simulink model "equ_diff"  (R2014a)
settings: Solver=ode45  StartTime=0.0  StopTime=10  RelTol=1e-3
values from neighbouring files (symbols this model uses):
  g = 9.81    [boucle_ferme.m]    (also in commande.m; var.m = 9.8)
  lp = 0.3    [boucle_ferme.m]    (also in commande.m; var.m = 0.2)
  mc = 0.5    [boucle_ferme.m]    (also in commande.m; var.m = 0.1)
  mp = 0.2    [boucle_ferme.m]    (also in commande.m; var.m)
settings Model: Creator=yassin  LastModifiedBy=yassin
settings DebuggingCC: UnderspecifiedInitializationDetection=Classic  StateNameClashWarn=warning

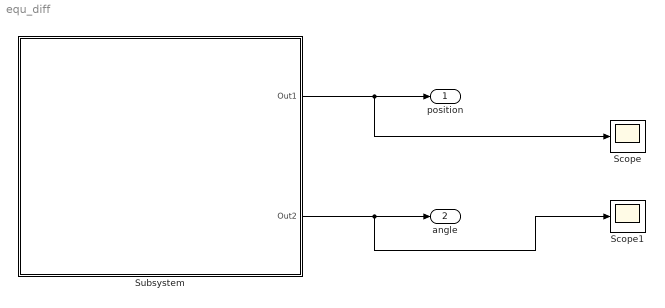
== system equ_diff ==
  Scope : Scope
  Scope1 : Scope
  Subsystem : Subsystem
  position : Outport
  angle : Outport  Port=2
  wires:
  Subsystem/1(Out1) -> Scope/1, position/1
  Subsystem/2(Out2) -> Scope1/1, angle/1

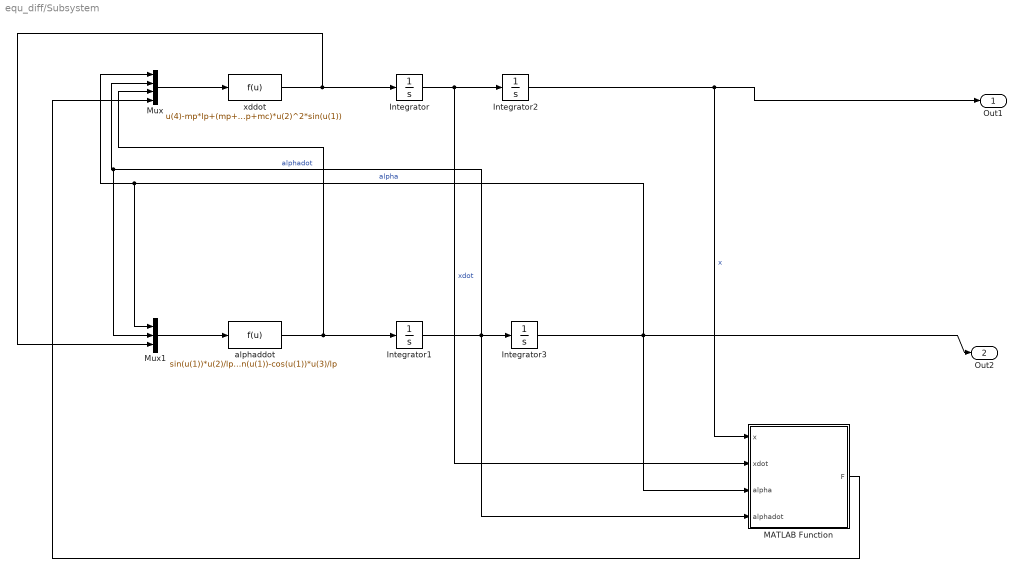
== system equ_diff/Subsystem ==
  Integrator : Integrator
  Integrator1 : Integrator
  Integrator2 : Integrator
  Integrator3 : Integrator  InitialCondition=0.5
  MATLAB Function : MATLAB Function  TreatAsAtomicUnit=on
  Mux : Mux
  Mux1 : Mux  Inputs=3
  alphaddot : Fcn  Expr=sin(u(1))*u(2)/lp+g/lp*sin(u(1))-cos(u(1))*u(3)/lp
  xddot : Fcn  Expr=u(4)-mp*lp+(mp+mc)*u(3)*cos(u(1))-mp*lp/(mp+mc)*u(2)^2*sin(u(1))
  Out1 : Outport
  Out2 : Outport  Port=2
  wires:
  Integrator1/1 -> MATLAB Function/4(alphadot), Mux1/2, Mux/2, Integrator3/1  "alphadot"
  Integrator/1 -> MATLAB Function/2(xdot), Integrator2/1  "xdot"
  Integrator3/1 -> MATLAB Function/3(alpha), Out2/1, Mux1/1, Mux/1  "alpha"
  Mux/1 -> xddot/1
  Integrator2/1 -> Out1/1, MATLAB Function/1(x)  "x"
  Mux1/1 -> alphaddot/1
  alphaddot/1 -> Mux/3, Integrator1/1
  MATLAB Function/1(F) -> Mux/4
  xddot/1 -> Mux1/3, Integrator/1

== matlab function equ_diff/Subsystem/MATLAB Function ==
  data: x input; F output; xdot input; alpha input; alphadot input
function F = fcn(x,xdot,alpha,alphadot)
%#codegen

F = -[-10.0000  -85.0299  -18.9566  -17.6289]*[x,alpha,xdot,alphadot]';
return
end
